simulink model "TST_EnumTypes"  (Simulink 10.0)
settings: Solver=FixedStepDiscrete  StartTime=0.0  StopTime=10.0  FixedStep=0.02  RelTol=1e-3  EnableMultiTasking=on
undefined symbols (not defined in the file): DIL_VmmGsFcsCommandsMessage_LatApModeCmd, DIL_VmmGsFcsCommandsMessage_LongApModeCmd
settings Model: Creator=kharthforeign  LastModifiedBy=unknown
settings DataIOCC: LimitDataPoints=on  SignalLoggingSaveFormat=ModelDataLogs  SaveOutput=off  SignalLogging=off  SaveTime=off
settings OptimizationCC: BlockReduction=off  ConditionallyExecuteInputs=off  OptimizeBlockIOStorage=off  BufferReuse=off  GlobalBufferReuse=off  ExpressionFolding=off  ExpressionDepthLimit=2147483647  LocalBlockOutputs=off  InitFltsAndDblsToZero=on  OptimizeDataStoreBuffers=off  BusAssignmentInplaceUpdate=off
settings DebuggingCC: SolverPrmCheckMsg=warning  FcnCallInpInsideContextMsg=warning  StateNameClashWarn=warning
settings SFSimCC: SimParseCustomCode=off
settings GRTTargetCC: GeneratePreprocessorConditionals=Disable all
settings ConfigComp: CovExternalEMLEnable=off

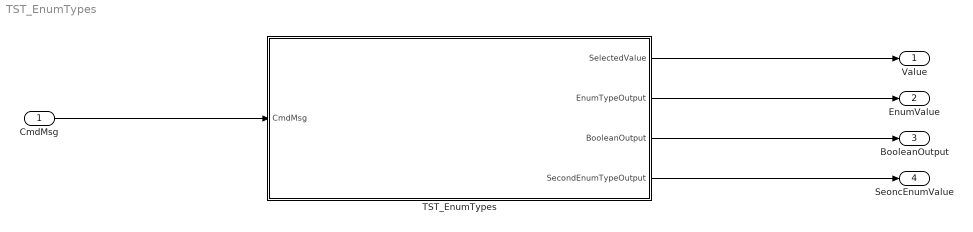
== system TST_EnumTypes ==
  CmdMsg : Inport  OutDataTypeStr=Bus: DIL_VmmGsFcsCommandsMessage_Data  BusOutputAsStruct=on
  TST_EnumTypes : Subsystem  TreatAsAtomicUnit=on
  Value : Outport  OutDataTypeStr=double  PortDimensions=1
  EnumValue : Outport  Port=2  OutDataTypeStr=Enum: DIL_VmmGsFcsCommandsMessage_LongApModeCmd  PortDimensions=1
  BooleanOutput : Outport  Port=3  OutDataTypeStr=boolean  PortDimensions=1
  SeoncEnumValue : Outport  Port=4  OutDataTypeStr=Enum: DIL_VmmGsFcsCommandsMessage_LongApModeCmd  PortDimensions=1
  wires:
  CmdMsg/1 -> TST_EnumTypes/1(CmdMsg)
  TST_EnumTypes/1(SelectedValue) -> Value/1
  TST_EnumTypes/2(EnumTypeOutput) -> EnumValue/1
  TST_EnumTypes/3(BooleanOutput) -> BooleanOutput/1
  TST_EnumTypes/4(SecondEnumTypeOutput) -> SeoncEnumValue/1

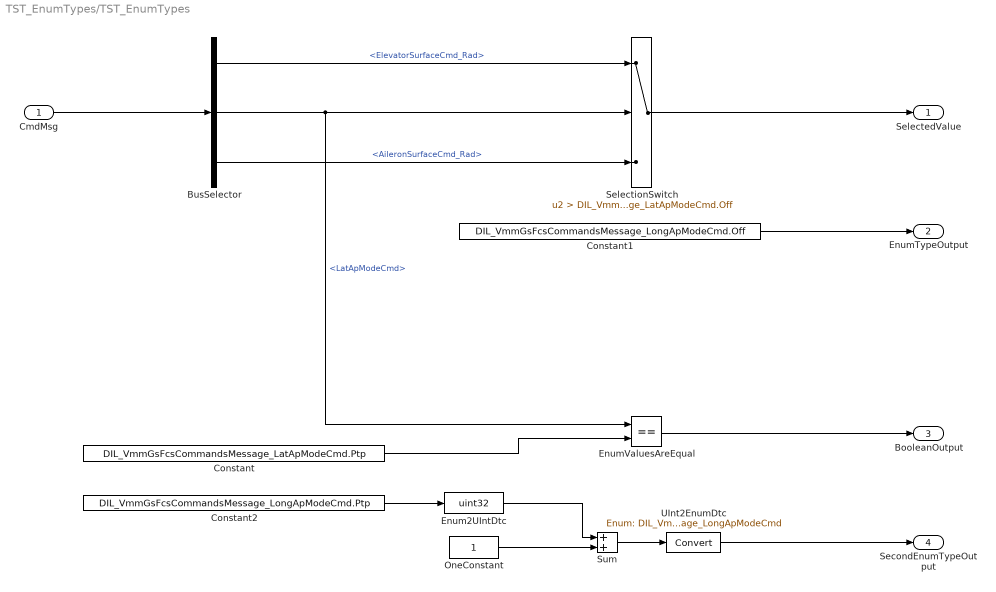
== system TST_EnumTypes/TST_EnumTypes ==
  CmdMsg : Inport  OutDataTypeStr=Bus: DIL_VmmGsFcsCommandsMessage_Data
  BusSelector : BusSelector  OutputSignals=ElevatorSurfaceCmd_Rad,LatApModeCmd,AileronSurfaceCmd_Rad
  Constant : Constant  Value=DIL_VmmGsFcsCommandsMessage_LatApModeCmd.Ptp  OutDataTypeStr=Enum: DIL_VmmGsFcsCommandsMessage_LatApModeCmd
  Constant1 : Constant  Value=DIL_VmmGsFcsCommandsMessage_LongApModeCmd.Off
  Constant2 : Constant  Value=DIL_VmmGsFcsCommandsMessage_LongApModeCmd.Ptp
  Enum2UIntDtc : DataTypeConversion  OutDataTypeStr=uint32
  EnumValuesAreEqual : RelationalOperator  Operator===  OutDataTypeStr=boolean  RndMeth=Nearest
  OneConstant : Constant  OutDataTypeStr=uint32
  SelectionSwitch : Switch  Criteria=u2 > Threshold  Threshold=DIL_VmmGsFcsCommandsMessage_LatApModeCmd.Off
  Sum : Sum
  UInt2EnumDtc : DataTypeConversion  OutDataTypeStr=Enum: DIL_VmmGsFcsCommandsMessage_LongApModeCmd
  SelectedValue : Outport  OutDataTypeStr=double  PortDimensions=1
  EnumTypeOutput : Outport  Port=2  OutDataTypeStr=Enum: DIL_VmmGsFcsCommandsMessage_LongApModeCmd  PortDimensions=1
  BooleanOutput : Outport  Port=3  OutDataTypeStr=boolean  PortDimensions=1
  SecondEnumTypeOutput : Outport  Port=4  OutDataTypeStr=Enum: DIL_VmmGsFcsCommandsMessage_LongApModeCmd  PortDimensions=1
  wires:
  CmdMsg/1 -> BusSelector/1
  SelectionSwitch/1 -> SelectedValue/1
  BusSelector/1 -> SelectionSwitch/1  "<ElevatorSurfaceCmd_Rad>"
  BusSelector/3 -> SelectionSwitch/3  "<AileronSurfaceCmd_Rad>"
  BusSelector/2 -> SelectionSwitch/2, EnumValuesAreEqual/1  "<LatApModeCmd>"
  Constant1/1 -> EnumTypeOutput/1
  EnumValuesAreEqual/1 -> BooleanOutput/1
  Constant/1 -> EnumValuesAreEqual/2
  Constant2/1 -> Enum2UIntDtc/1
  Enum2UIntDtc/1 -> Sum/1
  Sum/1 -> UInt2EnumDtc/1
  UInt2EnumDtc/1 -> SecondEnumTypeOutput/1
  OneConstant/1 -> Sum/2
